simulink model "AmpOp_Matlab_Versao_R2018b"  (R2018b)
settings: Solver=ode45  StartTime=0.0  StopTime=2  FixedStep=0.01  RelTol=1e-3
libraries: powerlib x15, simulink x1
settings Model: Creator=user  LastModifiedBy=user

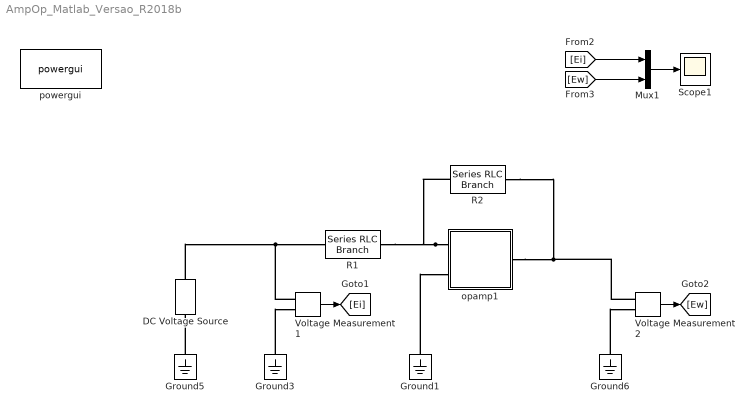
== system AmpOp_Matlab_Versao_R2018b ==
  DC Voltage Source : powerlib/Electrical Sources/DC Voltage Source  Amplitude=1  Measurements=None
  Ground{1,3,5..6} (4 alike) : powerlib/Elements/Ground  LConnTagsString=a
  Mux1 : Mux  Inputs=2
  R1 : powerlib/Elements/Series RLC Branch  LConnTagsString=__new0  RConnTagsString=__new0  BranchType=R  Resistance=50e3  Inductance=1e-3  SetiL0=off  InitialCurrent=0  Capacitance=1e-6  Setx0=off  InitialVoltage=0  Measurements=None
  R2 : powerlib/Elements/Series RLC Branch  LConnTagsString=__new0  RConnTagsString=__new0  BranchType=R  Resistance=100e3  Inductance=1e-3  SetiL0=off  InitialCurrent=0  Capacitance=1e-6  Setx0=off  InitialVoltage=0  Measurements=None
  Scope1 : Scope
  Voltage Measurement1 : powerlib/Measurements/Voltage Measurement  PhasorSimulation=off  OutputType=Complex  PSBequivalent=0
  Voltage Measurement2 : powerlib/Measurements/Voltage Measurement  PhasorSimulation=off  OutputType=Complex  PSBequivalent=0
  opamp1 : Subsystem  mask(Opamp){Ri=1e7, Ro=100, A=200000, U1=12, U2=-12}
      mask prompts: Ri "Input Resistance"; Ro "Output Resistance"; A "Open loop amplification"; U1 "Upper limit supply voltage"; U2 "Lower limit supply voltage"
      mask Display:
      | plot([10 20 30 40], [10 12 14 16],[10 20 30 40], [22 20 18 16],[10 10],[10 22])
      | text(10,13.4,'+')
      | text(10,21,'_')
  powergui : powerlib/powergui  Priority=1  SimulationMode=Discrete  SampleTime=1e-5  frequency=60  Iterations=50  frequencyindice=0  Pbase=100e6  ErrMax=1e-4  UnitsV=kV  UnitsW=MW  buscounter=0  FunctionMessages=off  echomessages=off  EnableUseOfTLC=off  CurrentSourceSwitches=off  DisableSnubberDevices=off  DisableRonSwitches=off  DisableVfSwitches=off  DisplayEquations=off  SolverType=Tustin/Backward Euler (TBE)  Interpol=off  ExternalGateDelay=off  methode=off  Ts=100  x0status=blocks  SPID=off  SwTol=0  HookPort=off  RestoreLinks=warning  ResistiveCurrentMeasurement=off  Frange=[0:2:500]  Ylog=off  Xlog=on  ShowGrid=off  save=off  variable=ZData  structure=0  ZoomFFT=off  StartTime=0.0  cycles=1  DisplayStyle=1  fundamental=60  FreqAxis=off  MaxFrequency=1000  frequencyindicesteady=1  RmsSteady=1  display=off
  wires:
  Voltage Measurement1/1 -> [Ei]
  Voltage Measurement2/1 -> [Ew]
  Mux1/1 -> Scope1/1
  [Ei] -> Mux1/1
  [Ew] -> Mux1/2
  connections:
  opamp1/LConn1 -- R2/LConn1 -- R1/RConn1
  Ground1/LConn1 -- opamp1/LConn2
  opamp1/RConn1 -- R2/RConn1 -- Voltage Measurement2/LConn1
  Ground3/LConn1 -- Voltage Measurement1/LConn2
  Voltage Measurement1/LConn1 -- DC Voltage Source/RConn1 -- R1/LConn1
  Ground5/LConn1 -- DC Voltage Source/LConn1
  Ground6/LConn1 -- Voltage Measurement2/LConn2

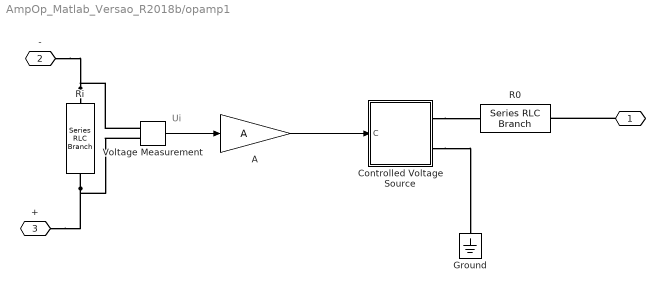
== system AmpOp_Matlab_Versao_R2018b/opamp1 ==
  note: Ui
  A : Gain  Gain=A
  Controlled Voltage Source : Subsystem
  Ground : powerlib/Elements/Ground  LConnTagsString=a
  R0 : powerlib/Elements/Series RLC Branch  LConnTagsString=__new0  RConnTagsString=__new0  BranchType=R  Resistance=Ro  Inductance=1.0  SetiL0=off  InitialCurrent=0  Capacitance=1.0  Setx0=off  InitialVoltage=0  Measurements=None
  Ri : powerlib/Elements/Series RLC Branch  LConnTagsString=__new0  RConnTagsString=__new0  BranchType=R  Resistance=Ri  Inductance=1.0  SetiL0=off  InitialCurrent=0  Capacitance=1.0  Setx0=off  InitialVoltage=0  Measurements=None
  Voltage Measurement : powerlib/Measurements/Voltage Measurement  PhasorSimulation=off  OutputType=Complex  PSBequivalent=0
  " " : PMIOPort  Side=Right
  - : PMIOPort  Port=2  Side=Left
  + : PMIOPort  Port=3  Side=Left
  wires:
  A/1 -> Controlled Voltage Source/1(C)
  Voltage Measurement/1 -> A/1
  connections:
  Controlled Voltage Source/RConn2 -- Ground/LConn1
  Ri/RConn1 -- Voltage Measurement/LConn2 -- +/RConn1
  Ri/LConn1 -- Voltage Measurement/LConn1 -- -/RConn1
  Controlled Voltage Source/RConn1 -- R0/RConn1
  " "/RConn1 -- R0/LConn1

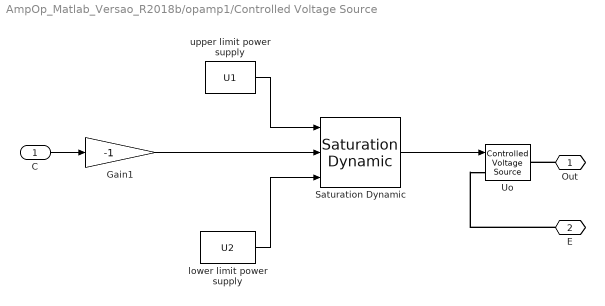
== system AmpOp_Matlab_Versao_R2018b/opamp1/Controlled Voltage Source ==
  C : Inport
  Gain1 : Gain  Gain=-1
  Saturation Dynamic : simulink/Discontinuities/Saturation Dynamic  OutMin=[]  OutMax=[]  OutDataTypeStr=Inherit: Same as second input  OutDataType=fixdt(1, 16)  OutScaling=2^-10  DoSatur=off
  Uo : powerlib/Electrical Sources/Controlled Voltage Source  Initialize=off  Source_Type=AC  Amplitude=0  Phase=0  Frequency=0  Measurements=None
  lower limit power supply : Constant  Value=U2
  upper limit power supply : Constant  Value=U1
  Out : PMIOPort  Side=Right
  E : PMIOPort  Port=2  Side=Right
  wires:
  Gain1/1 -> Saturation Dynamic/2
  lower limit power supply/1 -> Saturation Dynamic/3
  upper limit power supply/1 -> Saturation Dynamic/1
  C/1 -> Gain1/1
  Saturation Dynamic/1 -> Uo/1
  connections:
  Out/RConn1 -- Uo/RConn1
  E/RConn1 -- Uo/LConn1
